simulink model "problem_8"  (R2020b)
settings: Solver=VariableStepAuto  StartTime=0.0  StopTime=10.0  RelTol=1e-3
settings Model: Creator=hp  LastModifiedBy=hp

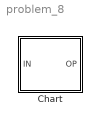
== system problem_8 ==
  Chart : Stateflow chart  TreatAsAtomicUnit=on

== stateflow chart problem_8/Chart ==
  state Shift_Control [parallel]
    en:
    settings: executionOrder=1
    state Ideal
    state DOWNSHIFT
    state UPSHIFT
    (default) -> Ideal
    Ideal -> UPSHIFT : [IN=IN+1]{send(UPSHIFT,}
  state LIFT_CONTROL [parallel]
    settings: executionOrder=2
    state FLOOR_1
      en:
      OP=1;
    state FLOOR_2
      en:
      OP=2;
    state FLOOR_3
      en:
      OP=3;
    state FLOOR_4
      en:
      OP=4;
    state FLOOR_5
      en:
      OP=5;
    (default) -> FLOOR_1
    FLOOR_4 -> FLOOR_5 [order 1] : UP
    FLOOR_3 -> FLOOR_4 [order 1] : UP
    FLOOR_2 -> FLOOR_3 [order 1] : UP
    FLOOR_1 -> FLOOR_2 : UP
    FLOOR_2 -> FLOOR_1 [order 2] : DOWN
    FLOOR_3 -> FLOOR_2 [order 2] : DOWN
    FLOOR_5 -> FLOOR_4 : DOWN
    FLOOR_4 -> FLOOR_3 [order 2] : DOWN
  (default) -> Shift_Control
  data: IN input; OP output
  events: UP local FUNCTION_CALL_EVENT; DOWN local FUNCTION_CALL_EVENT
